simulink model "leo_chukwuezi_sim_3pt5_sipro"  (R2024b)
settings: Solver=VariableStepAuto  StartTime=0.0  StopTime=8  RelTol=1e-3
model workspace (MAT data in the model file):
  Ki = 2.7
values from neighbouring files (symbols this model uses):
  G = 1    [leo_chukwuezi_sipro_lab2.m]
  KD = 0.75    [leo_chukwuezi_sipro_lab2.m]
  KI = 2.70    (= 2.7)    [leo_chukwuezi_sipro_lab2.m]
  KP = 1.25    [leo_chukwuezi_sipro_lab2.m]
  Ts = ts    (= 0.1)    [leo_chukwuezi_sipro_lab2.m]
  wo = 2    [leo_chukwuezi_sipro_lab2.m]
undefined symbols (not defined in the file or in its folder): dend, dspblkCoreblockFVToolHelper, gcbh, numd
settings Model: Creator=DELL E7320  LastModifiedBy=DELL E7320

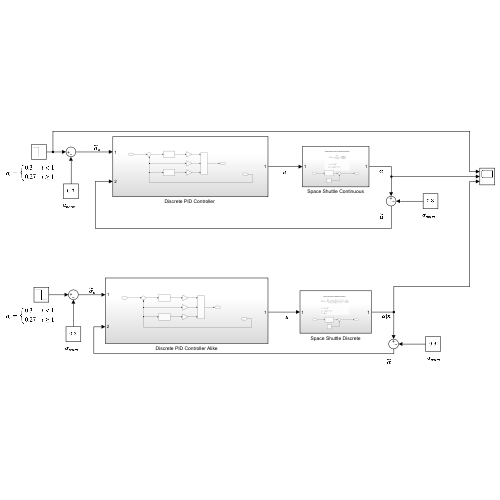
[thumbnail: Simulink's stored preview of the top-level diagram]
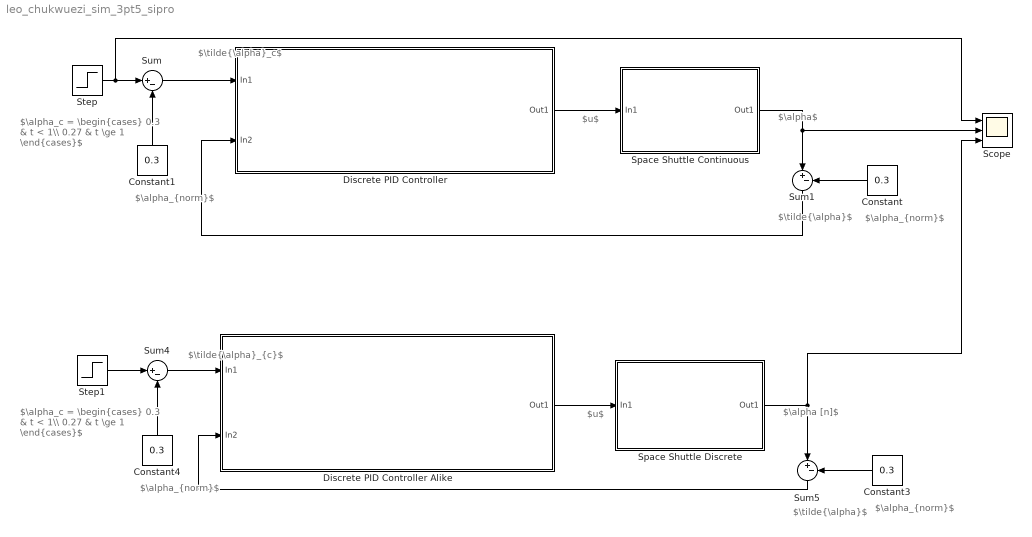
== system leo_chukwuezi_sim_3pt5_sipro ==
  note: $\alpha_{norm}$
  note: $\tilde{\alpha}$
  note: $\alpha$
  note: $u$
  note: $\alpha_c = \begin{cases} 0.3 & t < 1\\ 0.27 & t \ge 1 \end{cases}$
  note: $\alpha_{norm}$
  note: $\alpha_{norm}$
  note: $\alpha_{norm}$
  note: $\tilde{\alpha}$
  note: $\tilde{\alpha}_c$
  note: $\tilde{\alpha}_{c}$
  note: $\alpha_c = \begin{cases} 0.3 & t < 1\\ 0.27 & t \ge 1 \end{cases}$
  note: $u$
  note: $\alpha [n]$
  Constant{,1,3..4} (4 alike) : Constant  Value=0.3
  "Discrete PID Controller " : Subsystem
  Discrete PID Controller Alike : Subsystem
  Scope : Scope  NumInputPorts=3
  Space Shuttle Continuous : Subsystem
  Space Shuttle Discrete : Subsystem
  Step : Step  Before=0.3  After=0.27  SampleTime=0.1
  Step1 : Step  Before=0.3  After=0.27  SampleTime=0.1
  Sum{,1,4..5} (4 alike) : Sum  Inputs=|+-
  wires:
  Step/1 -> Scope/1, Sum/1
  Constant/1 -> Sum1/2
  Constant1/1 -> Sum/2
  Constant4/1 -> Sum4/2
  Constant3/1 -> Sum5/2
  Step1/1 -> Sum4/1
  Space Shuttle Continuous/1(Out1) -> Sum1/1, Scope/2
  Space Shuttle Discrete/1(Out1) -> Sum5/1, Scope/3
  Sum/1 -> "Discrete PID Controller "/1(In1)
  Sum1/1 -> "Discrete PID Controller "/2(In2)
  "Discrete PID Controller "/1(Out1) -> Space Shuttle Continuous/1(In1)
  Sum4/1 -> Discrete PID Controller Alike/1(In1)
  Sum5/1 -> Discrete PID Controller Alike/2(In2)
  Discrete PID Controller Alike/1(Out1) -> Space Shuttle Discrete/1(In1)

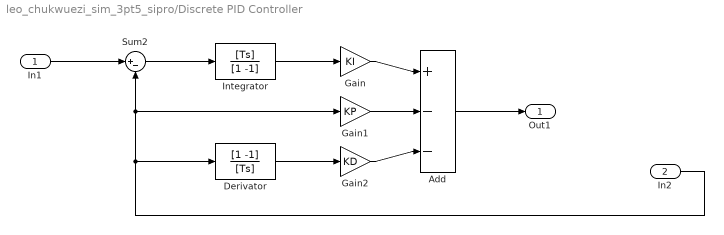
== system leo_chukwuezi_sim_3pt5_sipro/Discrete PID Controller  ==
  In1 : Inport
  In2 : Inport  Port=2
  Add : Sum  Inputs=+|-|-
  Derivator : DiscreteFilter  LoadFcn=dspblkCoreblockFVToolHelper(gcbh,'load');  Numerator=[1 -1]  Denominator=[Ts]
      settings: CopyFcn=dspblkCoreblockFVToolHelper(gcbh,'copy');  DeleteFcn=dspblkCoreblockFVToolHelper(gcbh,'close');  ModelCloseFcn=dspblkCoreblockFVToolHelper(gcbh,'close');  PreSaveFcn=dspblkCoreblockFVToolHelper(gcbh,'presave');  PostSaveFcn=dspblkCoreblockFVToolHelper(gcbh,'postsave');  CloseFcn=dspblkCoreblockFVToolHelper(gcbh,'close');
  Gain : Gain  Gain=KI
  Gain1 : Gain  Gain=KP
  Gain2 : Gain  Gain=KD
  Integrator : DiscreteFilter  LoadFcn=dspblkCoreblockFVToolHelper(gcbh,'load');  Numerator=[Ts]  Denominator=[1 -1]
      settings: CopyFcn=dspblkCoreblockFVToolHelper(gcbh,'copy');  DeleteFcn=dspblkCoreblockFVToolHelper(gcbh,'close');  ModelCloseFcn=dspblkCoreblockFVToolHelper(gcbh,'close');  PreSaveFcn=dspblkCoreblockFVToolHelper(gcbh,'presave');  PostSaveFcn=dspblkCoreblockFVToolHelper(gcbh,'postsave');  CloseFcn=dspblkCoreblockFVToolHelper(gcbh,'close');
  Sum2 : Sum  Inputs=|+-
  Out1 : Outport
  wires:
  In1/1 -> Sum2/1
  Integrator/1 -> Gain/1
  In2/1 -> Derivator/1, Gain1/1, Sum2/2
  Gain2/1 -> Add/3
  Gain/1 -> Add/1
  Derivator/1 -> Gain2/1
  Sum2/1 -> Integrator/1
  Gain1/1 -> Add/2
  Add/1 -> Out1/1

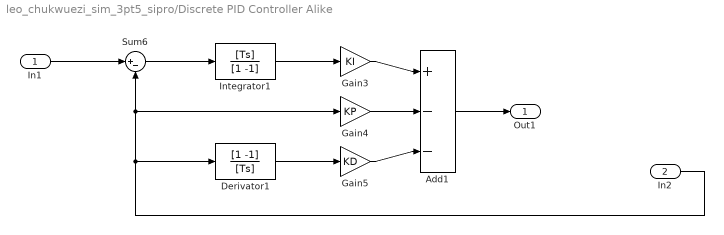
== system leo_chukwuezi_sim_3pt5_sipro/Discrete PID Controller Alike ==
  In1 : Inport
  In2 : Inport  Port=2
  Add1 : Sum  Inputs=+|-|-
  Derivator1 : DiscreteFilter  LoadFcn=dspblkCoreblockFVToolHelper(gcbh,'load');  Numerator=[1 -1]  Denominator=[Ts]
      settings: CopyFcn=dspblkCoreblockFVToolHelper(gcbh,'copy');  DeleteFcn=dspblkCoreblockFVToolHelper(gcbh,'close');  ModelCloseFcn=dspblkCoreblockFVToolHelper(gcbh,'close');  PreSaveFcn=dspblkCoreblockFVToolHelper(gcbh,'presave');  PostSaveFcn=dspblkCoreblockFVToolHelper(gcbh,'postsave');  CloseFcn=dspblkCoreblockFVToolHelper(gcbh,'close');
  Gain3 : Gain  Gain=KI
  Gain4 : Gain  Gain=KP
  Gain5 : Gain  Gain=KD
  Integrator1 : DiscreteFilter  LoadFcn=dspblkCoreblockFVToolHelper(gcbh,'load');  Numerator=[Ts]  Denominator=[1 -1]
      settings: CopyFcn=dspblkCoreblockFVToolHelper(gcbh,'copy');  DeleteFcn=dspblkCoreblockFVToolHelper(gcbh,'close');  ModelCloseFcn=dspblkCoreblockFVToolHelper(gcbh,'close');  PreSaveFcn=dspblkCoreblockFVToolHelper(gcbh,'presave');  PostSaveFcn=dspblkCoreblockFVToolHelper(gcbh,'postsave');  CloseFcn=dspblkCoreblockFVToolHelper(gcbh,'close');
  Sum6 : Sum  Inputs=|+-
  Out1 : Outport
  wires:
  In2/1 -> Derivator1/1, Gain4/1, Sum6/2
  Gain4/1 -> Add1/2
  Derivator1/1 -> Gain5/1
  Gain3/1 -> Add1/1
  Integrator1/1 -> Gain3/1
  Sum6/1 -> Integrator1/1
  Gain5/1 -> Add1/3
  Add1/1 -> Out1/1
  In1/1 -> Sum6/1

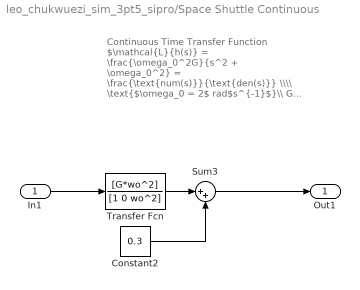
== system leo_chukwuezi_sim_3pt5_sipro/Space Shuttle Continuous ==
  note: Continuous Time Transfer Function
      |
      | $\mathcal{L}{h(s)} = \frac{\omega_0^2G}{s^2 + \omega_0^2} = \frac{\text{num(s)}}{\text{den(s)}} \\\\ \text{$\omega_0 = 2$ rad$s^{-1}$}\\ G = 1\, \text{rad.}N^{-1}.m^{-1}\\ %Ts = 0.1\,s$
  In1 : Inport
  Constant2 : Constant  Value=0.3
  Sum3 : Sum  Inputs=|++
  Transfer Fcn : TransferFcn  Numerator=[G*wo^2]  Denominator=[1 0 wo^2]
  Out1 : Outport
  wires:
  Transfer Fcn/1 -> Sum3/1
  In1/1 -> Transfer Fcn/1
  Sum3/1 -> Out1/1
  Constant2/1 -> Sum3/2

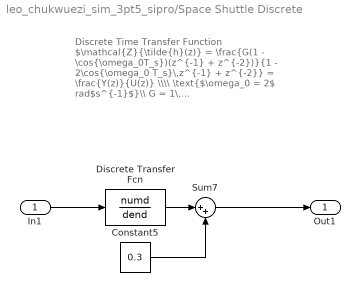
== system leo_chukwuezi_sim_3pt5_sipro/Space Shuttle Discrete ==
  note: Discrete Time Transfer Function
      |
      | $\mathcal{Z}{\tilde{h}(z)} = \frac{G(1 - \cos{\omega_0T_s})(z^{-1} + z^{-2})}{1 - 2\cos{\omega_0 T_s}\,z^{-1} + z^{-2}} = \frac{Y(z)}{U(z)} \\\\ \text{$\omega_0 = 2$ rad$s^{-1}$}\\ G = 1\, \text{rad.}N^{-1}.m^{-1}\\ T_s = 0.1\,s$
  In1 : Inport
  Constant5 : Constant  Value=0.3
  Discrete Transfer Fcn : DiscreteTransferFcn  LoadFcn=dspblkCoreblockFVToolHelper(gcbh,'load');  Numerator=numd  Denominator=dend
      settings: CopyFcn=dspblkCoreblockFVToolHelper(gcbh,'copy');  DeleteFcn=dspblkCoreblockFVToolHelper(gcbh,'close');  ModelCloseFcn=dspblkCoreblockFVToolHelper(gcbh,'close');  PreSaveFcn=dspblkCoreblockFVToolHelper(gcbh,'presave');  PostSaveFcn=dspblkCoreblockFVToolHelper(gcbh,'postsave');  CloseFcn=dspblkCoreblockFVToolHelper(gcbh,'close');
  Sum7 : Sum  Inputs=|++
  Out1 : Outport
  wires:
  Discrete Transfer Fcn/1 -> Sum7/1
  Constant5/1 -> Sum7/2
  In1/1 -> Discrete Transfer Fcn/1
  Sum7/1 -> Out1/1
